simulink model "model"  (R2020b)
settings: Solver=VariableStepAuto  StartTime=0.0  StopTime=10  FixedStep=0.1  RelTol=1e-3
StopFcn:
  | Plotter;
libraries: simulink x1
settings Model: EnablePacing=on  Creator=berkg  LastModifiedBy=volkan

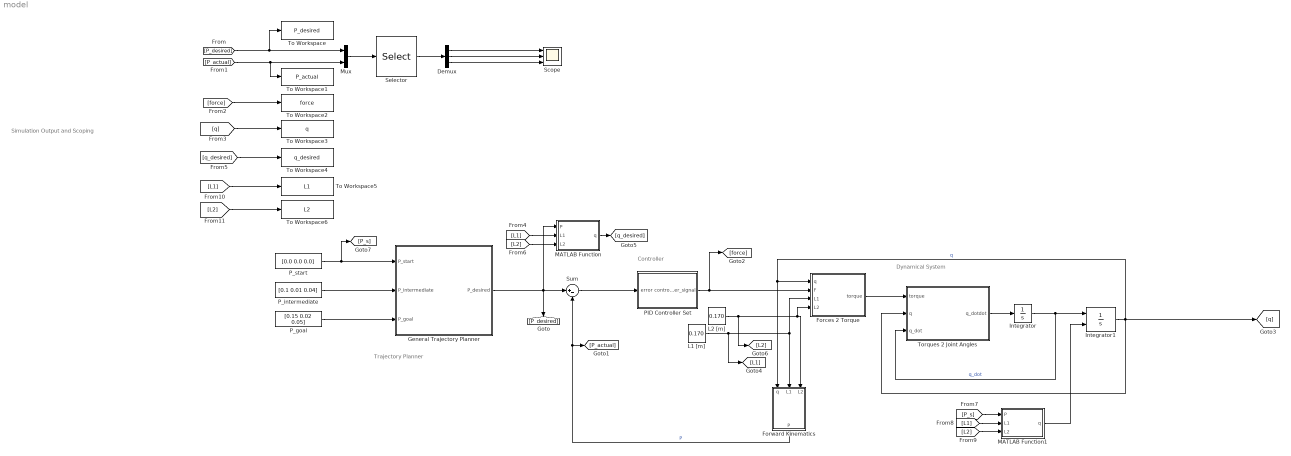
== system model ==
  note: Simulation Output
      | and Scoping
  note: Trajectory Planner
  note: Dynamical System
  note: Controller
  Demux : Demux  Outputs=3
  Forces 2 Torque : MATLAB Function  TreatAsAtomicUnit=on
  Forward Kinematics : MATLAB Function  TreatAsAtomicUnit=on
  General Trajectory Planner : Subsystem
  Integrator : Integrator  InitialCondition=[0 0 0]
  Integrator1 : Integrator  InitialConditionSource=external  InitialCondition=[0 0 0]
  L1 [m] : Constant  Value=0.170
  L2 [m] : Constant  Value=0.170
  MATLAB Function : MATLAB Function  TreatAsAtomicUnit=on
  MATLAB Function1 : MATLAB Function  TreatAsAtomicUnit=on
  Mux : Mux  Inputs=2
  PID Controller Set : Subsystem
  P_goal : Constant  Value=[0.15 0.02 0.05]
  P_intermediate : Constant  Value=[0.1 0.01 0.04]
  P_start : Constant  Value=[0.0 0.0 0.0]
  Scope : Scope  NumInputPorts=3
  Selector : Selector  InputPortWidth=6  IndexOptions=Index vector (dialog)  Indices=[[1,4], [2,5], [3,6]]  OutputSizes=1
  Sum : Sum  Inputs=|+-
  To Workspace : ToWorkspace  VariableName=P_desired  SampleTime=-1
      settings: Save2DSignal=2-D array (concatenate along first dimension)
  To Workspace1 : ToWorkspace  VariableName=P_actual  SampleTime=-1
      settings: Save2DSignal=2-D array (concatenate along first dimension)
  To Workspace2 : ToWorkspace  VariableName=force  SampleTime=-1
      settings: Save2DSignal=2-D array (concatenate along first dimension)
  To Workspace3 : ToWorkspace  VariableName=q  SampleTime=-1
      settings: Save2DSignal=2-D array (concatenate along first dimension)
  To Workspace4 : ToWorkspace  VariableName=q_desired  SampleTime=-1
      settings: Save2DSignal=2-D array (concatenate along first dimension)
  To Workspace5 : ToWorkspace  VariableName=L1  SampleTime=-1
      settings: Save2DSignal=2-D array (concatenate along first dimension)
  To Workspace6 : ToWorkspace  VariableName=L2  SampleTime=-1
      settings: Save2DSignal=2-D array (concatenate along first dimension)
  "Torques 2 Joint Angles " : MATLAB Function  TreatAsAtomicUnit=on
  wires:
  "Torques 2 Joint Angles "/1(q_dotdot) -> Integrator/1
  Integrator/1 -> Integrator1/1, "Torques 2 Joint Angles "/3(q_dot)  "q_dot"
  Integrator1/1 -> [q], "Torques 2 Joint Angles "/2(q), Forward Kinematics/1(q), Forces 2 Torque/1(q)  "q"
  L1 [m]/1 -> Forces 2 Torque/3(L1), Forward Kinematics/2(L1), [L1]
  L2 [m]/1 -> [L2], Forces 2 Torque/4(L2), Forward Kinematics/3(L2)
  P_intermediate/1 -> General Trajectory Planner/2(P_intermediate)
  P_goal/1 -> General Trajectory Planner/3(P_goal)
  P_start/1 -> [P_s], General Trajectory Planner/1(P_start)
  PID Controller Set/1(controller_signal) -> Forces 2 Torque/2(F), [force]
  Forward Kinematics/1(P) -> Sum/2, [P_actual]  "P"
  General Trajectory Planner/1(P_desired) -> MATLAB Function/1(P), Sum/1, [P_desired]
  Sum/1 -> PID Controller Set/1(error)
  [P_actual] -> To Workspace1/1, Mux/2
  Mux/1 -> Selector/1
  Selector/1 -> Demux/1
  Demux/1 -> Scope/1
  Demux/2 -> Scope/2
  Demux/3 -> Scope/3
  [P_desired] -> To Workspace/1, Mux/1
  [force] -> To Workspace2/1
  [q] -> To Workspace3/1
  [L1] -> MATLAB Function/2(L1)
  MATLAB Function/1(q) -> [q_desired]
  [q_desired] -> To Workspace4/1
  [L2] -> MATLAB Function/3(L2)
  [P_s] -> MATLAB Function1/1(P)
  [L1] -> MATLAB Function1/2(L1)
  [L2] -> MATLAB Function1/3(L2)
  MATLAB Function1/1(q) -> Integrator1/2
  Forces 2 Torque/1(torque) -> "Torques 2 Joint Angles "/1(torque)
  [L1] -> To Workspace5/1
  [L2] -> To Workspace6/1

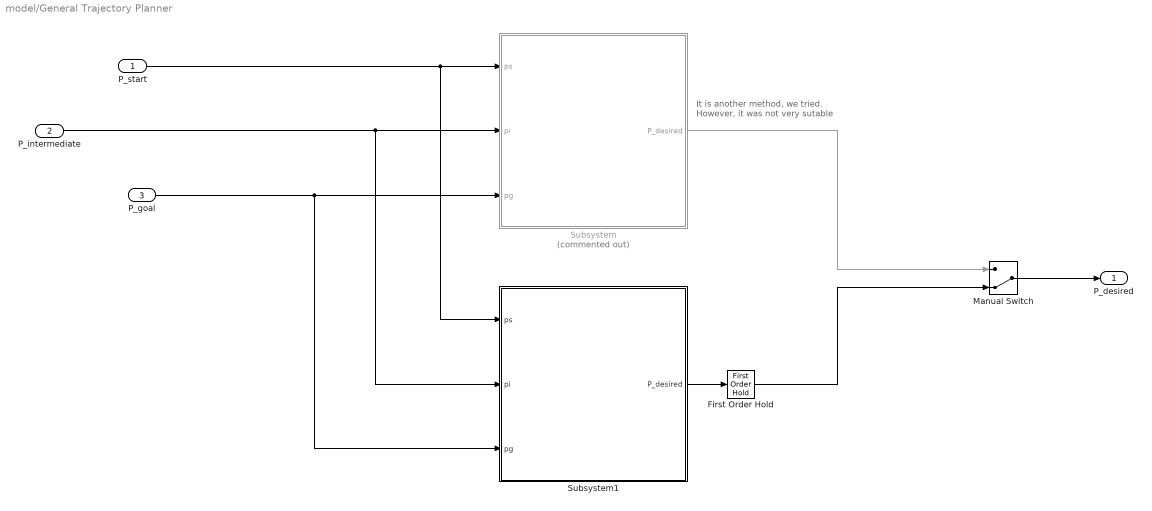
== system model/General Trajectory Planner ==
  note: It is another method, we tried.
      | However, it was not very sutable
  P_start : Inport
  P_intermediate : Inport  Port=2
  P_goal : Inport  Port=3
  First Order Hold : FirstOrderHold  ErrorTolerance=inf
  Manual Switch : ManualSwitch  CurrentSetting=0
  Subsystem : Subsystem  Commented=on
  Subsystem1 : Subsystem
  P_desired : Outport
  wires:
  P_start/1 -> Subsystem1/1(ps), Subsystem/1(ps)
  P_intermediate/1 -> Subsystem1/2(pi), Subsystem/2(pi)
  P_goal/1 -> Subsystem1/3(pg), Subsystem/3(pg)
  Subsystem/1(P_desired) -> Manual Switch/1
  Subsystem1/1(P_desired) -> First Order Hold/1
  Manual Switch/1 -> P_desired/1
  First Order Hold/1 -> Manual Switch/2

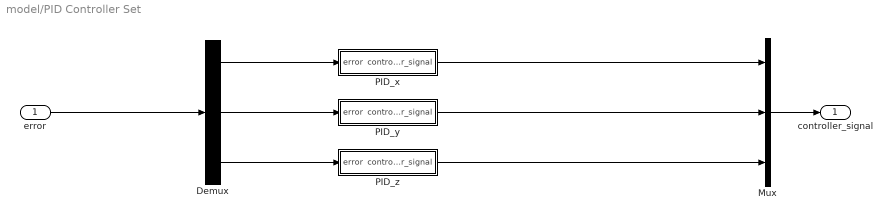
== system model/PID Controller Set ==
  error : Inport
  Demux : Demux  Outputs=3
  Mux : Mux  Inputs=3
  PID_x : Subsystem
  PID_y : Subsystem
  PID_z : Subsystem
  controller_signal : Outport
  wires:
  PID_x/1(controller_signal) -> Mux/1
  PID_z/1(controller_signal) -> Mux/3
  PID_y/1(controller_signal) -> Mux/2
  error/1 -> Demux/1
  Demux/3 -> PID_z/1(error)
  Demux/2 -> PID_y/1(error)
  Demux/1 -> PID_x/1(error)
  Mux/1 -> controller_signal/1

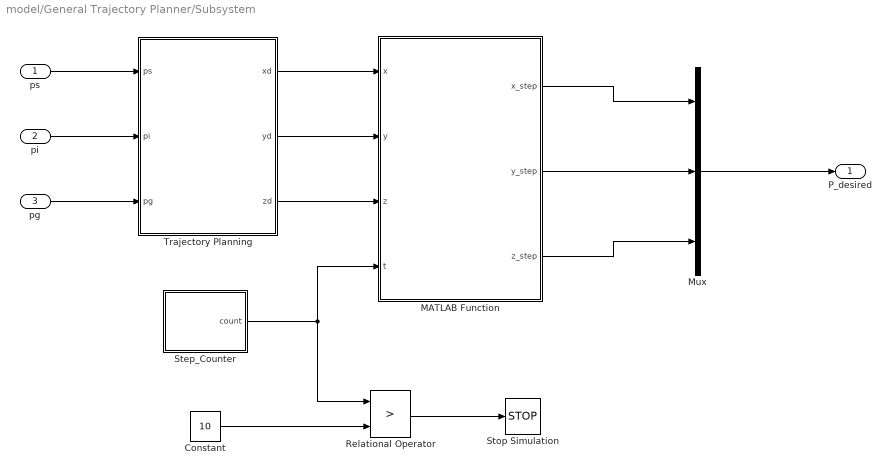
== system model/General Trajectory Planner/Subsystem ==
  ps : Inport
  pi : Inport  Port=2
  pg : Inport  Port=3
  Constant : Constant  Value=10
  MATLAB Function : MATLAB Function  TreatAsAtomicUnit=on
  Mux : Mux  Inputs=3
  Relational Operator : RelationalOperator  Operator=>  OutDataTypeStr=boolean  RndMeth=Simplest
  Step_Counter : Subsystem
  Stop Simulation : Stop
  Trajectory Planning : MATLAB Function  TreatAsAtomicUnit=on  SystemSampleTime=0.1
  P_desired : Outport
  wires:
  Step_Counter/1(count) -> MATLAB Function/4(t), Relational Operator/1
  pi/1 -> Trajectory Planning/2(pi)
  Trajectory Planning/2(yd) -> MATLAB Function/2(y)
  MATLAB Function/2(y_step) -> Mux/2
  Trajectory Planning/3(zd) -> MATLAB Function/3(z)
  Trajectory Planning/1(xd) -> MATLAB Function/1(x)
  MATLAB Function/3(z_step) -> Mux/3
  pg/1 -> Trajectory Planning/3(pg)
  MATLAB Function/1(x_step) -> Mux/1
  Constant/1 -> Relational Operator/2
  Mux/1 -> P_desired/1
  Relational Operator/1 -> Stop Simulation/1
  ps/1 -> Trajectory Planning/1(ps)

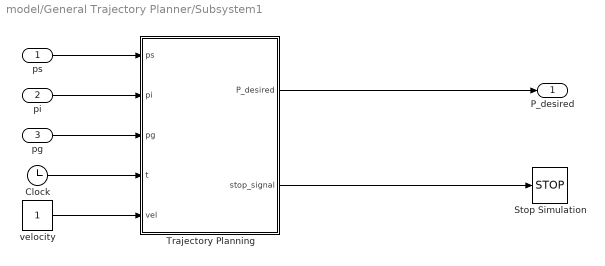
== system model/General Trajectory Planner/Subsystem1 ==
  ps : Inport
  pi : Inport  Port=2
  pg : Inport  Port=3
  Clock : Clock
  Stop Simulation : Stop
  Trajectory Planning : MATLAB Function  TreatAsAtomicUnit=on  SystemSampleTime=0.1
  velocity : Constant
  P_desired : Outport
  wires:
  ps/1 -> Trajectory Planning/1(ps)
  pg/1 -> Trajectory Planning/3(pg)
  pi/1 -> Trajectory Planning/2(pi)
  velocity/1 -> Trajectory Planning/5(vel)
  Clock/1 -> Trajectory Planning/4(t)
  Trajectory Planning/2(stop_signal) -> Stop Simulation/1
  Trajectory Planning/1(P_desired) -> P_desired/1

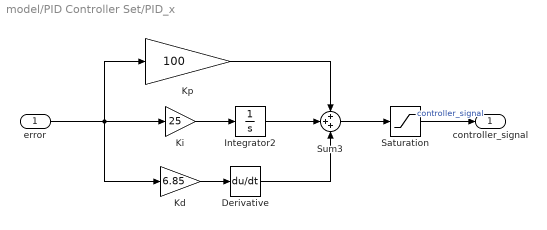
== system model/PID Controller Set/PID_x ==
  error : Inport
  Derivative : Derivative  CoefficientInTFapproximation=0
  Integrator2 : Integrator
  Kd : Gain  Gain=6.85
  Ki : Gain  Gain=25
  Kp : Gain  Gain=100
  Saturation : Saturate  UpperLimit=1  LowerLimit=-1
  Sum3 : Sum  Inputs=+++
  controller_signal : Outport
  wires:
  Ki/1 -> Integrator2/1
  error/1 -> Kd/1, Kp/1, Ki/1
  Derivative/1 -> Sum3/3
  Integrator2/1 -> Sum3/2
  Kd/1 -> Derivative/1
  Kp/1 -> Sum3/1
  Sum3/1 -> Saturation/1
  Saturation/1 -> controller_signal/1  "controller_signal"

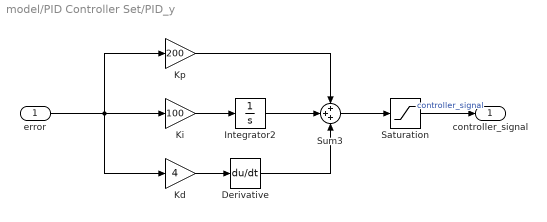
== system model/PID Controller Set/PID_y ==
  error : Inport
  Derivative : Derivative  CoefficientInTFapproximation=0
  Integrator2 : Integrator
  Kd : Gain  Gain=4
  Ki : Gain  Gain=100
  Kp : Gain  Gain=200
  Saturation : Saturate  UpperLimit=1  LowerLimit=-1
  Sum3 : Sum  Inputs=+++
  controller_signal : Outport
  wires:
  Ki/1 -> Integrator2/1
  error/1 -> Kd/1, Kp/1, Ki/1
  Derivative/1 -> Sum3/3
  Integrator2/1 -> Sum3/2
  Kd/1 -> Derivative/1
  Kp/1 -> Sum3/1
  Sum3/1 -> Saturation/1
  Saturation/1 -> controller_signal/1  "controller_signal"

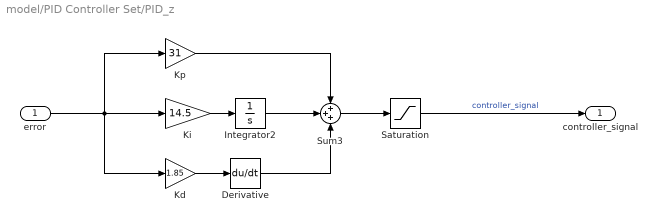
== system model/PID Controller Set/PID_z ==
  error : Inport
  Derivative : Derivative  CoefficientInTFapproximation=0
  Integrator2 : Integrator
  Kd : Gain  Gain=1.85
  Ki : Gain  Gain=14.5
  Kp : Gain  Gain=31
  Saturation : Saturate  UpperLimit=1  LowerLimit=-1
  Sum3 : Sum  Inputs=+++
  controller_signal : Outport
  wires:
  Ki/1 -> Integrator2/1
  error/1 -> Kd/1, Kp/1, Ki/1
  Derivative/1 -> Sum3/3
  Integrator2/1 -> Sum3/2
  Kd/1 -> Derivative/1
  Kp/1 -> Sum3/1
  Sum3/1 -> Saturation/1
  Saturation/1 -> controller_signal/1  "controller_signal"

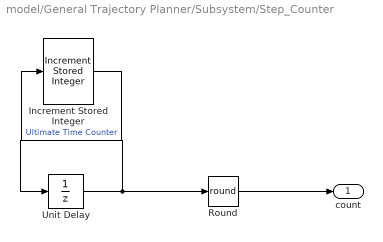
== system model/General Trajectory Planner/Subsystem/Step_Counter ==
  Increment Stored Integer : simulink/Additional Math & Discrete/Additional Math: Increment - Decrement/Increment Stored Integer
  Round : Rounding  Operator=round
  Unit Delay : UnitDelay  SampleTime=-1  HasFrameUpgradeWarning=on
  count : Outport
  wires:
  Unit Delay/1 -> Increment Stored Integer/1, Round/1  "Ultimate Time Counter"
  Increment Stored Integer/1 -> Unit Delay/1
  Round/1 -> count/1

== matlab function model/Forward Kinematics ==
  data: q input; P output; L1 input; L2 input
function P  = FK(q,L1,L2)
theta_1 = q(1); theta_2 = q(2); theta_3 = q(3);
Px = +sin(theta_1) * (L1 * cos(theta_2) + L2 * sin(theta_3));
Py = L2 - L2 * cos(theta_3) + L1 * sin(theta_2);
Pz = -L1 + cos(theta_1) * (L1*cos(theta_2) + L2 * sin(theta_3));

P = [Px, Py, Pz];

== matlab function model/Torques 2 Joint Angles  ==
  data: torque input; q input; q_dotdot output; q_dot input
function q_dotdot  = Robot_Dynamic(torque,q,q_dot)

q1 = q(1); q2 = q(2); q3 = q(3); 
q1d = q_dot(1); q2d = q_dot(2); q3d = q_dot(3); 

%% phantom premium 1.5 parameters
ma = 0.0202;%new
mc = 0.0249;%new
mbe = 0.2359;%new
mdf = 0.1906;
l1 = 0.215;%new
l2 = 0.170;
l3 = 0.0325;
l5 = -36.8e-3;
l6 = 52.7e-3;
g = 9.81;

%% moment of inertia params
Iaxx = 0.4864e-4;
Iayy = 0.001843e-4;
Iazz = 0.4864e-4;
Icxx = 0.959e-4;
Icyy = 0.959e-4;
Iczz = 0.0051e-4;
Ibexx = 11.09e-4;
Ibeyy = 10.06e-4;
Ibezz = 0.591e-4;
Idfxx = 7.11e-4;
Idfyy = 0.629e-4;
Idfzz = 6.246e-4;
Ibaseyy = 11.87e-4;

%% mass matrix components
m11 = (0.125*(4*Iayy+4*Iazz+8*Ibaseyy+4*Ibeyy+4*Ibezz+4*Icyy+4*Iczz+4*Idfyy+4*Idfzz+4*l1*l1*ma+l2*l2*ma+l1*l1*mc+4*l3*l3*mc)...
    +0.125*(4*Ibeyy-4*Ibezz+4*Icyy-4*Iczz+l1*l1*(4*ma+mc))*cos(2*q2)...
    +0.125*(4*Iayy-4*Iazz+4*Idfyy-4*Idfzz-l2*l2*ma-4*l3*l3*mc)*cos(2*q3)+l1*(l2*ma+l3*mc)*cos(q2)*sin(q3));
m22 = 0.25*(4*(Ibexx+Icxx+l1*l1*ma)+l1*l1*mc);
m23 = -0.5*l1*(l2*ma+l3*mc)*sin(q2-q3);
m32 = m23;
m33 = 0.25*(4*Iaxx+4*Idfxx+l2*l2*ma+4*l3*l3*mc);

M = [m11 0 0;
    0 m22 m23;
    0 m32 m33];


%% coriolis matrix components
c11 = 0.125*(-2*sin(q2)*((4*Ibeyy-4*Ibezz+4*Icyy-4*Iczz+4*l1*l1*ma+l1*l1*mc)*cos(q2)+2*l1*(l2*ma+l3*mc)*sin(q3))*q2d...
    +2*cos(q3)*(2*l1*(l2*ma+l3*mc)*cos(q2)+(-4*Iayy+4*Iazz-4*Idfyy+4*Idfzz+l2*l2*ma+4*l3*l3*mc)*sin(q3))*q3d);
c12 = -0.125*((4*Ibeyy-4*Ibezz+4*Icyy-4*Iczz+l1*l1*(4*ma+mc))*sin(2*q2)+4*l1*(l2*ma+l3*mc)*sin(q2)*sin(q3))*q1d;
c13 = -0.125*(-4*l1*(l2*ma+l3*mc)*cos(q2)*cos(q3)-(-4*Iayy+4*Iazz-4*Idfyy+4*Idfzz+l2*l2*ma+4*l3*l3*mc)*sin(2*q3))*q1d;
c21 = -c12;
c22 = 0;
c23 = 0.5*l1*(l2*ma+l3*mc)*cos(q2-q3)*q3d;
c31 = -c13;
c32 = 0.5*l1*(l2*ma+l3*mc)*cos(q2-q3)*q2d;
c33 = 0;

C = [c11 c12 c13;
    c21 c22 c23;
    c31 c32 c33];

%% gravity vector components
tg1 = 0;
tg2 = g*(l1*(ma+0.5*mc)+l5*mbe)*cos(q2);
tg3 = g*(0.5*l2*ma+l3*mc-l6*mdf)*sin(q3);


G = [0;
    tg2;
    tg3];

%% Forward Dynamic
q_dotdot = M\(torque-C*q_dot-G); % ==> M^(-1)*(torque-C-G)

== matlab function model/Forces 2 Torque ==
  data: q input; torque output; F input; L1 input; L2 input
function torque  = F2T(q,F,L1,L2)

%% Analytical Jacobian 
% Forward Differential Kinematics:
% If we take the derivative of the Forward Kinematic with respect to joint
% angle, we get the J(q)*q_dot:

theta_1 = q(1); theta_2 = q(2); theta_3 = q(3);
J = [L1*cos(theta_1)*cos(theta_2)+L2*sin(theta_3)*cos(theta_1) -L1*sin(theta_1)*sin(theta_2) L2*sin(theta_1)*cos(theta_3);
    0 L1*cos(theta_2) L2*sin(theta_3);
    -(L1*sin(theta_1)*cos(theta_2)+L2*sin(theta_1)*sin(theta_3)) -L1*sin(theta_2)*cos(theta_1) L2*cos(theta_1)*cos(theta_3)];

torque = J'*F;

== matlab function model/General Trajectory Planner/Subsystem/Trajectory Planning ==
  data: ps input; xd output; pi input; pg input; yd output; zd output
function [xd,yd,zd] = TP(ps,pi,pg)
% x = [ps(1) pi(1) pg(1)];
% y = [ps(2) pi(2) pg(2)];
% z = [ps(3) pi(3) pg(3)];
% h = line(x,y,z);
% xd = get(h,'XData'); yd = get(h,'YData'); zd = get(h,'ZData');
xd = [linspace(ps(1),pi(1),100),linspace(pi(1),pg(1),100)];
yd = [linspace(ps(2),pi(2),100),linspace(pi(2),pg(2),100)];
zd = [linspace(ps(3),pi(3),100),linspace(pi(3),pg(3),100)];    
%xd = get(h,'XData'); yd = get(h,'YData'); zd = get(h,'ZData');

== matlab function model/General Trajectory Planner/Subsystem/MATLAB Function ==
  data: x input; x_step output; y input; z input; y_step output; z_step output; t input
function [x_step,y_step, z_step] = slice_time(x,y,z, t)
t = t+1;
if t>200
    t = 200;
elseif t<1
        t = 1;
end
x_step = x(t);
y_step = y(t);
z_step = z(t);

== matlab function model/MATLAB Function ==
  data: P input; q output; L1 input; L2 input
function q  = IK(P, L1, L2)
Px = P(1); Py = P(2); Pz = P(3);
x = Px;
y = Py - L2;
z = Pz + L1;

% Elbow up - Base straight
q1_init = atan2(x,z);
r = sqrt(x^2+y^2+z^2);
L3 = sqrt(x^2+z^2);
q2_init = acos((L1^2+r^2-L2^2)/(2*L1*r)) + atan2(y,L3);
q3_init = acos((L1^2+L2^2-(x^2+y^2+z^2))/(2*L1*L2)) - pi/2 + q2_init;

q = [q1_init, q2_init, q3_init];

== matlab function model/General Trajectory Planner/Subsystem1/Trajectory Planning ==
  data: ps input; P_desired output; pi input; pg input; t input; vel input; stop_signal output
function [P_desired, stop_signal]  = TP(ps,pi,pg, t, vel)

stop_signal = 0;

% Representative velocity of the end effector
% from start to intermadiate point.
vel_s2i = (pi - ps) * vel;
% Required simulation time from start to 
% intermediate point.
t_s2i = norm(pi - ps) / norm(vel_s2i);

% Representative velocity of the end effector
% from start to intermadiate point.
vel_i2g = (pg - pi) * vel;
% Required simulation time from start to 
% intermediate point.
t_i2g = norm(pg - pi) / norm(vel_i2g);


% Total simulation time required for the
% path comletion
t_total = t_s2i + t_i2g;


% Motion propagation
if t <= t_s2i
     
    P_desired = ps + vel_s2i * t;
    
elseif (t_s2i < t) && (t <= t_total)
    
    P_desired = pi + vel_i2g * (t - t_s2i);
    
else
    
    P_desired = pg;
    % If motion ends, 
    % stop the simulation via ´stop_signal´
    stop_signal = 1;
    
end


end

== matlab function model/MATLAB Function1 ==
  data: P input; q output; L1 input; L2 input
function q  = IK(P, L1, L2)
Px = P(1); Py = P(2); Pz = P(3);
x = Px;
y = Py - L2;
z = Pz + L1;

% Elbow up - Base straight
q1 = atan2(x,z);
r = sqrt(x^2+y^2+z^2);
L3 = sqrt(x^2+z^2);
q2 = acos((L1^2+r^2-L2^2)/(2*L1*r)) + atan2(y,L3);
q3 = acos((L1^2+L2^2-(x^2+y^2+z^2))/(2*L1*L2)) - pi/2 + q2;

q = [q1, q2, q3];
